simulink model "parameters_identification"  (R2024a)
settings: Solver=VariableStepAuto  StartTime=0.0  StopTime=10.0  RelTol=1e-3
undefined symbols (not defined in the file or in its folder): Kcorrente
libraries: daqlib x1, slctrl_signal x1
settings Model: Creator=Guilherme  LastModifiedBy=Guilherme

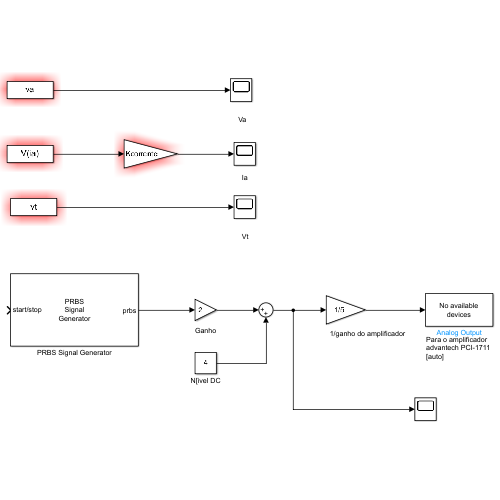
[thumbnail: Simulink's stored preview of the top-level diagram]
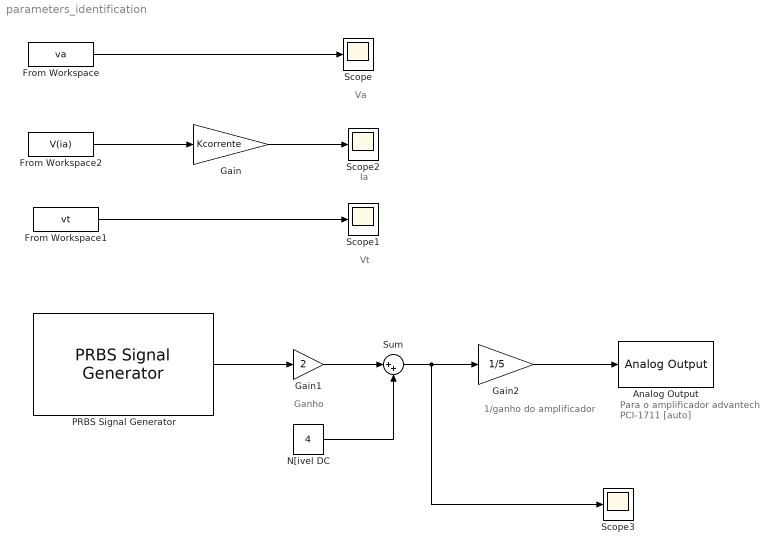
== system parameters_identification ==
  note: Para o amplificador advantech PCI-1711 [auto]
  note: 1/ganho do amplificador
  note: Ganho
  note: Ia
  note: Va
  note: Vt
  Analog Output : daqlib/Analog Output  DeviceMenu=(none)  Device=(none)  NChannelsSelected=1  NPorts=1 for all channels  SampleRate=0  ActualRate=0
  From Workspace : FromWorkspace  VariableName=va
  From Workspace1 : FromWorkspace  VariableName=vt
  From Workspace2 : FromWorkspace  VariableName=V(ia)
  Gain : Gain  Gain=Kcorrente
  Gain1 : Gain  Gain=2
  Gain2 : Gain  Gain=1/5
  N[ivel DC : Constant  Value=4
  PRBS Signal Generator : slctrl_signal/PRBS Signal Generator  DiscreteTs=0.1  BlockDataType=double  SignalSource=Block parameters  Frequencies=[0.5 1 2]  FreqUnits=rad/s  Amplitudes=1  NumOfFreq=3  NumOfPRBSPeriod=1  UseAutogenNumOfPRBSPeriod=off  PRBSSignalOrder=12  UseAutogenPRBSSignalOrder=off  UseExternalTs=off  CompiledTsChoice=InternalTs
      settings: LibrarySourceBlock=slctrlblks/Signal Generation/PRBS Signal Generator
  Scope{,1..3} (4 alike) : Scope
  Sum : Sum  Inputs=|++
  wires:
  From Workspace/1 -> Scope/1
  From Workspace1/1 -> Scope1/1
  From Workspace2/1 -> Gain/1
  Gain/1 -> Scope2/1
  Gain1/1 -> Sum/1
  N[ivel DC/1 -> Sum/2
  Sum/1 -> Scope3/1, Gain2/1
  Gain2/1 -> Analog Output/1
  PRBS Signal Generator/1 -> Gain1/1
